simulink model "fuzzy_dodawanie_mandani"  (R2024b)
settings: Solver=VariableStepDiscrete  StartTime=0.0  StopTime=10.0  MaxStep=0.01  RelTol=1e-3
libraries: fuzblock x3
settings Model: Creator=marci  LastModifiedBy=marci

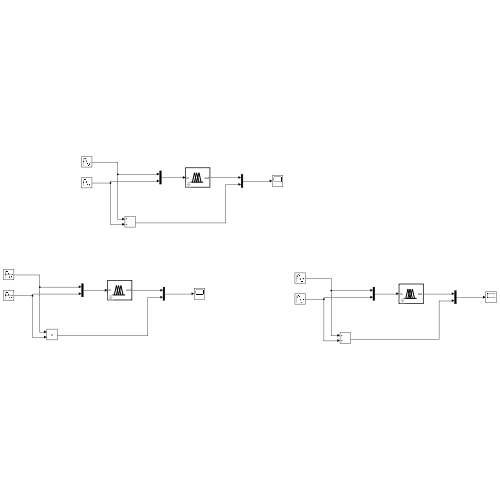
[thumbnail: Simulink's stored preview of the top-level diagram]
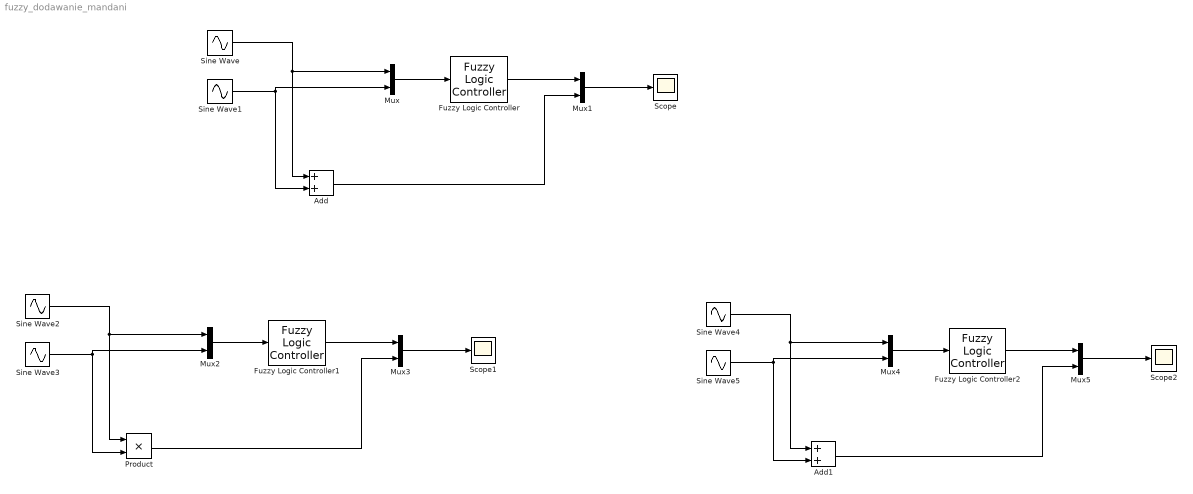
== system fuzzy_dodawanie_mandani ==
  Add : Sum
  Add1 : Sum
  Fuzzy Logic Controller : fuzblock/Fuzzy Logic  Controller  FIS=dodaj  OutputSampleNumber=101  DataType=double  FuzzifiedInputs=off  RuleFiringStrengths=off  RuleOutputs=off  AggregatedOutputs=off  SimulateUsing=Interpreted execution  OutOfRangeInputValueMessage=warning  NoRuleFiredMessage=warning  EmptyOutputFuzzySetMessage=warning
  Fuzzy Logic Controller1 : fuzblock/Fuzzy Logic  Controller  FIS=mnoz  OutputSampleNumber=101  DataType=double  FuzzifiedInputs=off  RuleFiringStrengths=off  RuleOutputs=off  AggregatedOutputs=off  SimulateUsing=Interpreted execution  OutOfRangeInputValueMessage=warning  NoRuleFiredMessage=warning  EmptyOutputFuzzySetMessage=warning
  Fuzzy Logic Controller2 : fuzblock/Fuzzy Logic  Controller  FIS=sugenotype1_dodawanie  OutputSampleNumber=101  DataType=double  FuzzifiedInputs=off  RuleFiringStrengths=off  RuleOutputs=off  AggregatedOutputs=off  SimulateUsing=Interpreted execution  OutOfRangeInputValueMessage=warning  NoRuleFiredMessage=warning  EmptyOutputFuzzySetMessage=warning
  Mux{,1..5} (6 alike) : Mux  Inputs=2
  Product : Product
  Scope : Scope
  Scope1 : Scope
  Scope2 : Scope
  Sine Wave : Sin  Amplitude=5  Bias=5  SampleTime=0
  Sine Wave1 : Sin  Amplitude=4  Bias=5  Frequency=3  SampleTime=0
  Sine Wave2 : Sin  Amplitude=5  Bias=5  SampleTime=0
  Sine Wave3 : Sin  Amplitude=4  Bias=5  Frequency=3  SampleTime=0
  Sine Wave4 : Sin  Amplitude=5  Bias=5  SampleTime=0
  Sine Wave5 : Sin  Amplitude=4  Bias=5  Frequency=3  SampleTime=0
  wires:
  Sine Wave/1 -> Mux/1, Add/1
  Sine Wave1/1 -> Add/2, Mux/2
  Mux/1 -> Fuzzy Logic Controller/1
  Fuzzy Logic Controller/1 -> Mux1/1
  Mux1/1 -> Scope/1
  Add/1 -> Mux1/2
  Product/1 -> Mux3/2
  Fuzzy Logic Controller1/1 -> Mux3/1
  Mux2/1 -> Fuzzy Logic Controller1/1
  Mux3/1 -> Scope1/1
  Sine Wave2/1 -> Product/1, Mux2/1
  Sine Wave3/1 -> Product/2, Mux2/2
  Mux4/1 -> Fuzzy Logic Controller2/1
  Sine Wave5/1 -> Add1/2, Mux4/2
  Add1/1 -> Mux5/2
  Mux5/1 -> Scope2/1
  Sine Wave4/1 -> Add1/1, Mux4/1
  Fuzzy Logic Controller2/1 -> Mux5/1
